simulink model "example_F27"  (R2016b)
settings: Solver=VariableStepAuto  StartTime=0.0  StopTime=30.0  RelTol=1e-3
PreLoadFcn:
  | k = 20;
  | m = 90;
  | C_viscous = 1;
  | C_drag = 1;
  | g = 9.81;
settings Model: Creator=training-ah  LastModifiedBy=training-ah

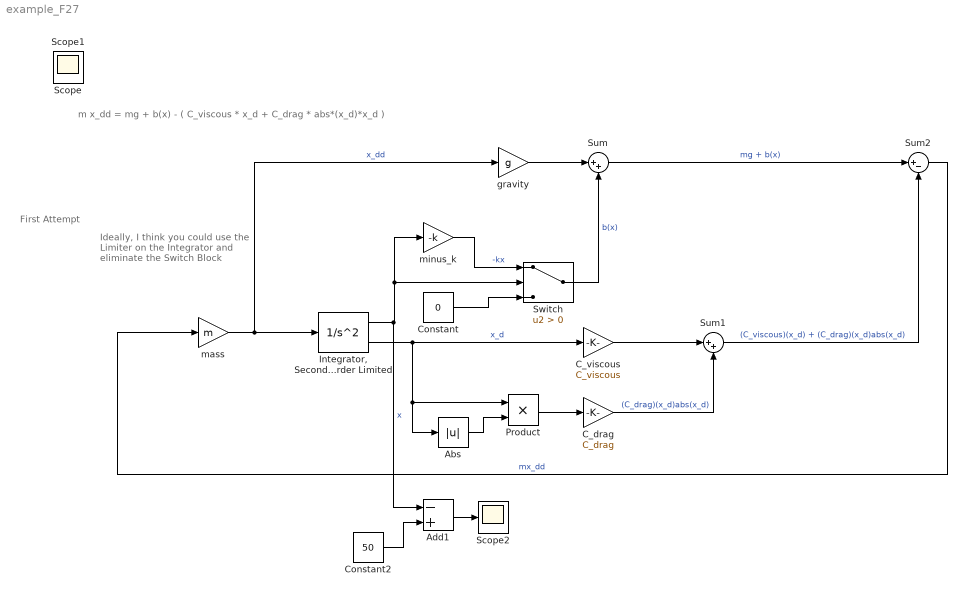
== system example_F27 ==
  note: Ideally, I think you could
      | use the Limiter on the Integrator
      | and eliminate the Switch Block
  note: First Attempt
  note: m x_dd = mg + b(x) - ( C_viscous * x_d + C_drag * abs*(x_d)*x_d )
  Abs : Abs
  Add1 : Sum  Inputs=-+
  C_drag : Gain  Gain=C_drag
  C_viscous : Gain  Gain=C_viscous
  Constant : Constant  Value=0
  Constant2 : Constant  Value=50
  "Integrator, Second-Order Limited" : SecondOrderIntegrator  ICX=-30.0  UpperLimitX=1  LowerLimitX=0
  Product : Product
  Scope2 : Scope
  Sum : Sum  Inputs=|++
  Sum1 : Sum  Inputs=|++
  Sum2 : Sum  Inputs=|+-
  Switch : Switch  Criteria=u2 > Threshold
  gravity : Gain  Gain=g
  mass : Gain  Gain=m
  minus_k : Gain  Gain=-k
  Scope : Scope
  Scope1 : Scope
  wires:
  mass/1 -> gravity/1, "Integrator, Second-Order Limited"/1  "x_dd"
  "Integrator, Second-Order Limited"/2 -> C_viscous/1, Abs/1, Product/1  "x_d"
  Sum2/1 -> mass/1  "mx_dd"
  gravity/1 -> Sum/1
  Sum/1 -> Sum2/1  "mg + b(x)"
  C_drag/1 -> Sum1/2  "(C_drag)(x_d)abs(x_d)"
  C_viscous/1 -> Sum1/1
  Abs/1 -> Product/2
  Product/1 -> C_drag/1
  Sum1/1 -> Sum2/2  "(C_viscous)(x_d) + (C_drag)(x_d)abs(x_d)"
  minus_k/1 -> Switch/1  "-kx"
  Constant/1 -> Switch/3
  Switch/1 -> Sum/2  "b(x)"
  "Integrator, Second-Order Limited"/1 -> Add1/1, minus_k/1, Switch/2  "x"
  Constant2/1 -> Add1/2
  Add1/1 -> Scope2/1
